simulink model "model_Differntial_equation"  (R2020b)
settings: Solver=VariableStepAuto  StartTime=0.0  StopTime=10.0  RelTol=1e-3
settings Model: Creator=Training  LastModifiedBy=Training

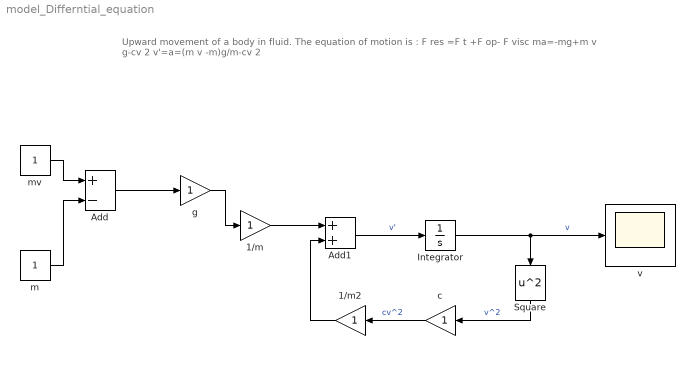
== system model_Differntial_equation ==
  note: Upward movement of a body in fluid.
      | The equation of motion is :
      | F res =F t +F op- F visc
      |
      | ma=-mg+m v g-cv 2
      |
      | v'=a=(m v -m)g/m-cv 2
  1/m : Gain
  1/m2 : Gain
  Add : Sum  Inputs=+-
  Add1 : Sum
  Integrator : Integrator
  Square : Math  Operator=square  SaturateOnIntegerOverflow=on
  c : Gain
  g : Gain
  m : Constant
  mv : Constant
  v : Scope
  wires:
  mv/1 -> Add/1
  m/1 -> Add/2
  Add/1 -> g/1
  Square/1 -> c/1  "v^2"
  g/1 -> 1/m/1
  Integrator/1 -> v/1, Square/1  "v"
  1/m/1 -> Add1/1
  c/1 -> 1/m2/1  "cv^2"
  1/m2/1 -> Add1/2
  Add1/1 -> Integrator/1  "v'"
